simulink model "Final"  (R2019a)
settings: Solver=VariableStepAuto  StartTime=0.0  StopTime=100  RelTol=1e-3
undefined symbols (not defined in the file): sigbuilder_block
settings Model: Creator=fjvel  LastModifiedBy=fjvel

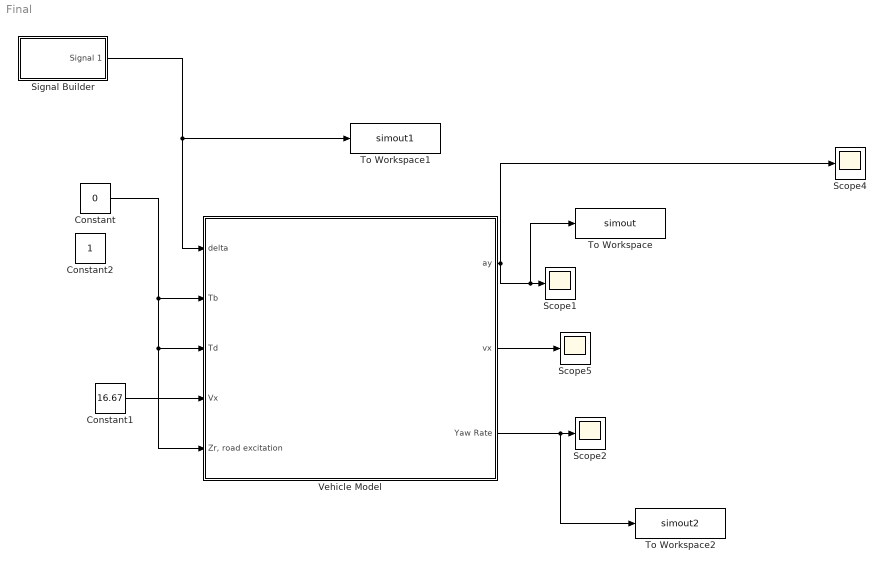
== system Final ==
  Constant : Constant  Value=0
  Constant1 : Constant  Value=16.67
  Constant2 : Constant
  Scope{1..2,4..5} (4 alike) : Scope
  Signal Builder : Subsystem  Tag=STV Subsys  LoadFcn=sigbuilder_block('load');  StartFcn=sigbuilder_block('start');  StopFcn=sigbuilder_block('stop');  ClipboardFcn=sigbuilder_block('clipboard');  mask(Sigbuilder block){tuvar=[0:10]}
      mask help: Simulink:masks:SigbuilderBlock_MD
      mask init:
      | if ~strcmp(get_param(bdroot(gcbh),'SimulationStatus'),'stopped') tuvar = sigbuilder_block('maskInit'); end
      settings: CopyFcn=sigbuilder_block('copy');  DeleteFcn=sigbuilder_block('delete');  ModelCloseFcn=sigbuilder_block('modelClose');  PreSaveFcn=sigbuilder_block('preSave');  PauseFcn=sigbuilder_block('pause');  ContinueFcn=sigbuilder_block('continue');  NameChangeFcn=sigbuilder_block('namechange');  OpenFcn=sigbuilder_block('open',[6 30 1012.5 447.75 ]);  CloseFcn=sigbuilder_block('close');
      mask Display: plot(0, 0, 100, 100,[2, 2, 32, 32, 2], [68, 8, 8, 68, 68],[32, 2], [38, 38], [32, 19, 2],[53, 60, 44], [32, 17, 17, 2],[16, 16, 31, 31]);txt = getActiveGroup(gcbh);text(2, 100, txt,'verticalAlignment', 'top');
  To Workspace : ToWorkspace  VariableName=simout  SaveFormat=Timeseries  SampleTime=-1
  To Workspace1 : ToWorkspace  VariableName=simout1  SaveFormat=Timeseries  SampleTime=-1
  To Workspace2 : ToWorkspace  VariableName=simout2  SaveFormat=Timeseries  SampleTime=-1
  Vehicle Model : Subsystem
  wires:
  Vehicle Model/2(vx) -> Scope5/1
  Constant/1 -> Vehicle Model/2(Tb), Vehicle Model/5("Zr, road excitation"), Vehicle Model/3(Td)
  Constant1/1 -> Vehicle Model/4("Vx ")
  Vehicle Model/1(ay) -> Scope4/1, To Workspace/1, Scope1/1
  Vehicle Model/3(Yaw Rate) -> To Workspace2/1, Scope2/1
  Signal Builder/1(Signal 1) -> Vehicle Model/1(delta), To Workspace1/1

== system Final/Signal Builder ==
  Demux : Demux  Tag=STV Demux  Outputs=1
  FromWs : FromWorkspace  Tag=STV FromWs  VariableName=tuvar  SampleTime=0
      SigBuilderData=|
      | common.afterFinalStr = 'Extrapolate'
      | common.sampleTime = 0
      | dataSet.timeRange = [0 10]
      | dataSet.name = 'Group 1'
      | sbobj.Groups.Name = 'Group 1'
      | sbobj.Groups.Signals.Name = 'Signal 1'
      | sbobj.Groups.Signals.XData = [0 3 3.03 3.47 3.5 10]
      | sbobj.Groups.Signals.YData = [0 0 0.042 0.042 0 0]
  Signal 1 : Outport  Tag=STV Outport
  wires:
  Demux/1 -> Signal 1/1
  FromWs/1 -> Demux/1

== system Final/Vehicle Model ==
  delta : Inport
  Tb : Inport  Port=2
  Td : Inport  Port=3
  "Vx " : Inport  Port=4  LockScale=on
  "Zr, road excitation" : Inport  Port=5
  Handling : Subsystem
  Scope : Scope
  Scope1 : Scope
  Scope2 : Scope
  Tire-Magic Formula Model : Subsystem
  Vertical Dynamics : Subsystem
  ay : Outport  VectorParamsAs1DForOutWhenUnconnected=on
  vx : Outport  Port=2  VectorParamsAs1DForOutWhenUnconnected=on
  Yaw Rate : Outport  Port=3  VectorParamsAs1DForOutWhenUnconnected=on
  wires:
  Handling/1(alpha_fl) -> Tire-Magic Formula Model/6(alpha_fl)
  Handling/2(alpha_fr) -> Tire-Magic Formula Model/8(alpha_fr)
  Handling/3(alpha_rl) -> Tire-Magic Formula Model/10(alpha_rl)
  Handling/4(alpha_rr) -> Tire-Magic Formula Model/12(alpha_rr)
  Handling/5(Sfl) -> Tire-Magic Formula Model/5(Sfl)
  Handling/6(Sfr) -> Tire-Magic Formula Model/7(Sfr)
  Handling/7(Srl) -> Tire-Magic Formula Model/9(Srl)
  Handling/8(Srr) -> Tire-Magic Formula Model/11(Srr)
  Tire-Magic Formula Model/1(Fxfl) -> Scope/1, Handling/2(Fxfl)
  Tire-Magic Formula Model/2(Fyfl) -> Scope1/1, Handling/3(Fyfl)
  Tire-Magic Formula Model/3(Fxfr) -> Handling/4(Fxfr)
  Tire-Magic Formula Model/4(Fyfr) -> Handling/5(Fyfr)
  Tire-Magic Formula Model/5(Fxrl) -> Handling/6(Fxrl)
  Tire-Magic Formula Model/6(Fyrl) -> Handling/7(Fyrl)
  Tire-Magic Formula Model/7(Fxrr) -> Handling/8(Fxrr)
  Tire-Magic Formula Model/8(Fyrr) -> Handling/9(Fyrr)
  Tire-Magic Formula Model/9(Mzfl) -> Scope2/1, Handling/10(Mzfl)
  Tire-Magic Formula Model/10(Mzfr) -> Handling/11(Mzfr)
  Tire-Magic Formula Model/11(Mzrl) -> Handling/12(Mzrl)
  Tire-Magic Formula Model/12(Mzrr) -> Handling/13(Mzrr)
  Td/1 -> Handling/14(Td)
  Tb/1 -> Handling/15(Tb)
  "Vx "/1 -> Handling/16(Vx)
  delta/1 -> Handling/1(delta)
  Handling/9(ax) -> Vertical Dynamics/1(ax)
  Handling/10(ay) -> ay/1, Vertical Dynamics/2(ay)
  Vertical Dynamics/1(Fzfl) -> Tire-Magic Formula Model/1(Fzfl)
  Vertical Dynamics/2(Fzfr) -> Tire-Magic Formula Model/2(Fzfr)
  Vertical Dynamics/3(Fzrl) -> Tire-Magic Formula Model/3("Fzrl ")
  Vertical Dynamics/4(Fzrr) -> Tire-Magic Formula Model/4(Fzrr)
  "Zr, road excitation"/1 -> Vertical Dynamics/3("Zr, road excitation")
  Handling/11("vx ") -> vx/1
  Handling/12(Yaw Rate) -> Yaw Rate/1

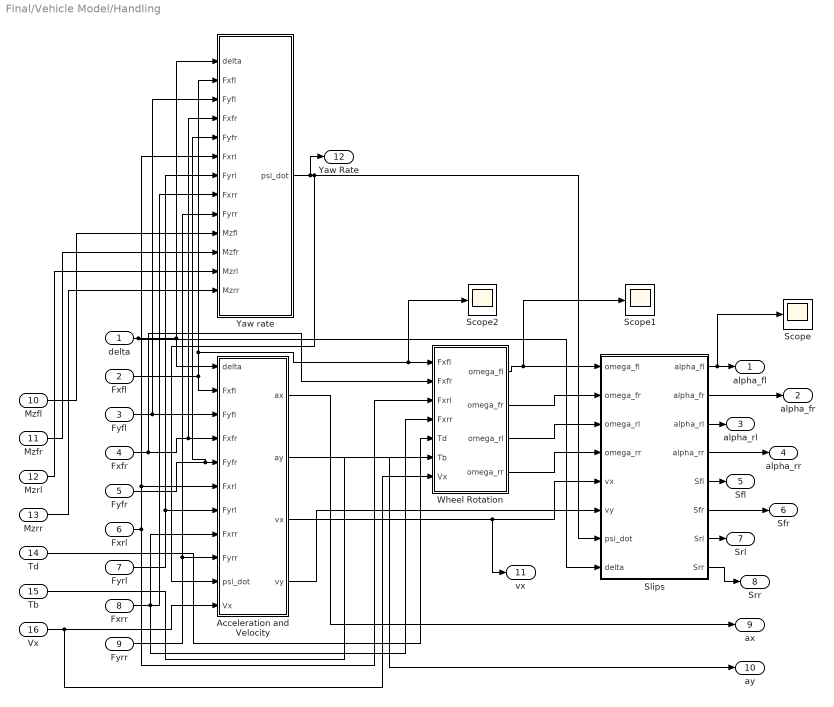
== system Final/Vehicle Model/Handling ==
  delta : Inport
  Fxfl : Inport  Port=2
  Fyfl : Inport  Port=3
  Fxfr : Inport  Port=4
  Fyfr : Inport  Port=5
  Fxrl : Inport  Port=6
  Fyrl : Inport  Port=7
  Fxrr : Inport  Port=8
  Fyrr : Inport  Port=9
  Mzfl : Inport  Port=10
  Mzfr : Inport  Port=11
  Mzrl : Inport  Port=12
  Mzrr : Inport  Port=13
  Td : Inport  Port=14
  Tb : Inport  Port=15
  Vx : Inport  Port=16
  "Acceleration and Velocity " : Subsystem
  Scope : Scope
  Scope1 : Scope
  Scope2 : Scope
  "Slips " : Subsystem
  Wheel Rotation : Subsystem
  Yaw rate : Subsystem
  alpha_fl : Outport
  alpha_fr : Outport  Port=2
  alpha_rl : Outport  Port=3
  alpha_rr : Outport  Port=4
  Sfl : Outport  Port=5
  Sfr : Outport  Port=6
  Srl : Outport  Port=7
  Srr : Outport  Port=8
  ax : Outport  Port=9
  ay : Outport  Port=10
  "vx " : Outport  Port=11  VectorParamsAs1DForOutWhenUnconnected=on
  Yaw Rate : Outport  Port=12  VectorParamsAs1DForOutWhenUnconnected=on
  wires:
  delta/1 -> "Slips "/8("delta "), Yaw rate/1(delta), "Acceleration and Velocity "/1(delta)
  Fxfl/1 -> Scope2/1, Wheel Rotation/1(Fxfl), Yaw rate/2(Fxfl), "Acceleration and Velocity "/2(Fxfl)
  Fyfl/1 -> Yaw rate/3(Fyfl), "Acceleration and Velocity "/3(Fyfl)
  Fxfr/1 -> Wheel Rotation/2(Fxfr), Yaw rate/4(Fxfr), "Acceleration and Velocity "/4(Fxfr)
  Fyfr/1 -> Yaw rate/5(Fyfr), "Acceleration and Velocity "/5(Fyfr)
  Fxrl/1 -> Wheel Rotation/3(Fxrl), Yaw rate/6(Fxrl), "Acceleration and Velocity "/6(Fxrl)
  Fyrl/1 -> Yaw rate/7(Fyrl), "Acceleration and Velocity "/7(Fyrl)
  Fxrr/1 -> Wheel Rotation/4(Fxrr), Yaw rate/8(Fxrr), "Acceleration and Velocity "/8(Fxrr)
  Fyrr/1 -> "Acceleration and Velocity "/9(Fyrr), Yaw rate/9(Fyrr)
  Vx/1 -> Wheel Rotation/7(Vx), "Acceleration and Velocity "/11(Vx)
  Mzfl/1 -> Yaw rate/10(Mzfl)
  Mzfr/1 -> Yaw rate/11(Mzfr)
  Mzrl/1 -> Yaw rate/12(Mzrl)
  Mzrr/1 -> Yaw rate/13(Mzrr)
  Yaw rate/1("psi_dot ") -> Yaw Rate/1, "Slips "/7(psi_dot), "Acceleration and Velocity "/10(psi_dot)
  Td/1 -> Wheel Rotation/5(Td)
  Tb/1 -> Wheel Rotation/6(Tb)
  Wheel Rotation/1(omega_fl) -> Scope1/1, "Slips "/1("omega_fl ")
  Wheel Rotation/2(omega_fr) -> "Slips "/2(omega_fr)
  Wheel Rotation/3(omega_rl) -> "Slips "/3(omega_rl)
  Wheel Rotation/4(omega_rr) -> "Slips "/4(omega_rr)
  "Acceleration and Velocity "/3(vx) -> "vx "/1, "Slips "/5(vx)
  "Acceleration and Velocity "/4(vy) -> "Slips "/6(vy)
  "Slips "/1(alpha_fl) -> Scope/1, alpha_fl/1
  "Slips "/2(alpha_fr) -> alpha_fr/1
  "Slips "/3(alpha_rl) -> alpha_rl/1
  "Slips "/4(alpha_rr) -> alpha_rr/1
  "Slips "/5("Sfl ") -> Sfl/1
  "Slips "/6(Sfr) -> Sfr/1
  "Slips "/7(Srl) -> Srl/1
  "Slips "/8(Srr) -> Srr/1
  "Acceleration and Velocity "/1(ax) -> ax/1
  "Acceleration and Velocity "/2(ay) -> ay/1

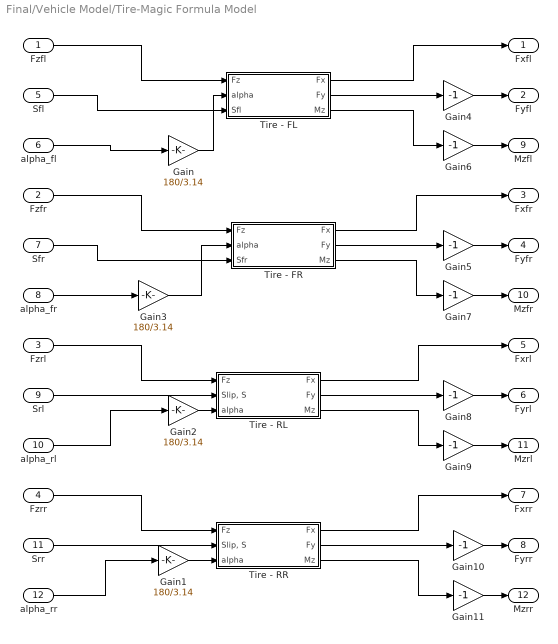
== system Final/Vehicle Model/Tire-Magic Formula Model ==
  Fzfl : Inport
  Fzfr : Inport  Port=2
  "Fzrl " : Inport  Port=3
  Fzrr : Inport  Port=4
  Sfl : Inport  Port=5
  alpha_fl : Inport  Port=6
  Sfr : Inport  Port=7
  alpha_fr : Inport  Port=8
  Srl : Inport  Port=9
  alpha_rl : Inport  Port=10
  Srr : Inport  Port=11
  alpha_rr : Inport  Port=12
  Gain{,1..3} (4 alike) : Gain  Gain=180/3.14
  Gain{4..11} (8 alike) : Gain  Gain=-1
  Tire - FL : Subsystem
  Tire - FR : Subsystem
  Tire - RL : Subsystem
  Tire - RR : Subsystem
  Fxfl : Outport
  Fyfl : Outport  Port=2
  Fxfr : Outport  Port=3
  Fyfr : Outport  Port=4
  Fxrl : Outport  Port=5
  Fyrl : Outport  Port=6
  Fxrr : Outport  Port=7
  Fyrr : Outport  Port=8
  Mzfl : Outport  Port=9
  Mzfr : Outport  Port=10
  Mzrl : Outport  Port=11
  Mzrr : Outport  Port=12
  wires:
  Fzfr/1 -> Tire - FR/1(Fz)
  Fzfl/1 -> Tire - FL/1(Fz)
  "Fzrl "/1 -> Tire - RL/1(Fz)
  Srl/1 -> Tire - RL/2("Slip, S")
  Fzrr/1 -> Tire - RR/1(Fz)
  Srr/1 -> Tire - RR/2("Slip, S")
  Tire - FL/1(Fx) -> Fxfl/1
  Tire - FL/2(Fy) -> Gain4/1
  Tire - FL/3(Mz) -> Gain6/1
  Tire - FR/2(Fy) -> Gain5/1
  Tire - FR/1(Fx) -> Fxfr/1
  Tire - FR/3(Mz) -> Gain7/1
  Tire - RL/1(Fx) -> Fxrl/1
  Tire - RL/2(Fy) -> Gain8/1
  Tire - RL/3(Mz) -> Gain9/1
  Tire - RR/1(Fx) -> Fxrr/1
  Tire - RR/2(Fy) -> Gain10/1
  Tire - RR/3(Mz) -> Gain11/1
  Sfl/1 -> Tire - FL/3("Sfl ")
  Sfr/1 -> Tire - FR/3(Sfr)
  alpha_fl/1 -> Gain/1
  Gain/1 -> Tire - FL/2(alpha)
  alpha_fr/1 -> Gain3/1
  Gain3/1 -> Tire - FR/2(alpha)
  Gain2/1 -> Tire - RL/3(alpha)
  Gain1/1 -> Tire - RR/3(alpha)
  alpha_rl/1 -> Gain2/1
  alpha_rr/1 -> Gain1/1
  Gain4/1 -> Fyfl/1
  Gain5/1 -> Fyfr/1
  Gain6/1 -> Mzfl/1
  Gain7/1 -> Mzfr/1
  Gain8/1 -> Fyrl/1
  Gain9/1 -> Mzrl/1
  Gain10/1 -> Fyrr/1
  Gain11/1 -> Mzrr/1

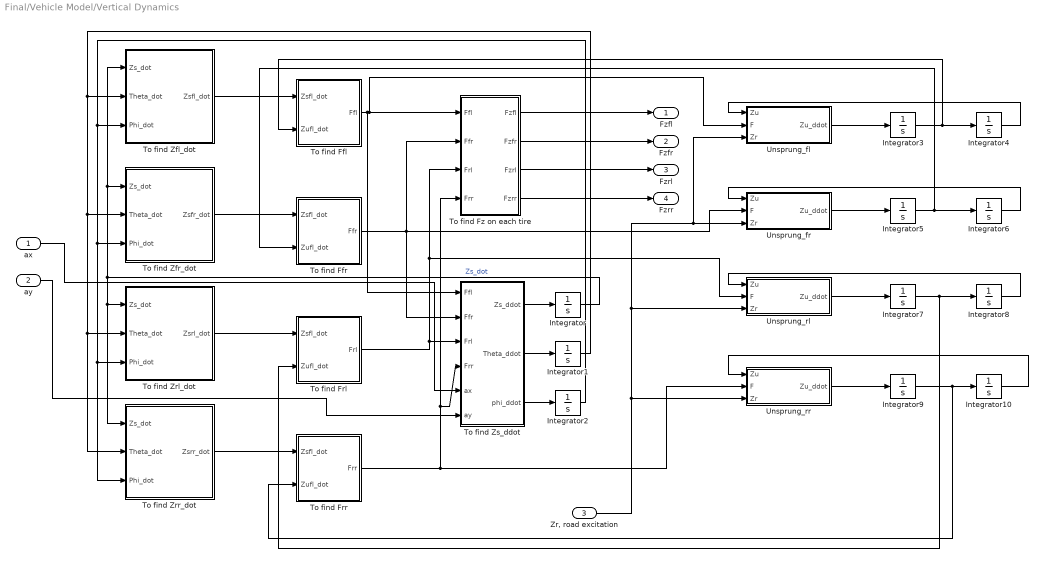
== system Final/Vehicle Model/Vertical Dynamics ==
  ax : Inport
  ay : Inport  Port=2
  "Zr, road excitation" : Inport  Port=3
  Integrator{,1..10} (11 alike) : Integrator
  "To find Ffl " : Subsystem
  To find Ffr : Subsystem
  To find Frl : Subsystem
  To find Frr : Subsystem
  To find Fz on each tire : Subsystem
  To find Zfl_dot : Subsystem
  To find Zfr_dot : Subsystem
  To find Zrl_dot : Subsystem
  To find Zrr_dot : Subsystem
  To find Zs_ddot : Subsystem
  Unsprung_fl : Subsystem
  Unsprung_fr : Subsystem
  Unsprung_rl : Subsystem
  Unsprung_rr : Subsystem
  Fzfl : Outport
  Fzfr : Outport  Port=2
  Fzrl : Outport  Port=3
  Fzrr : Outport  Port=4
  wires:
  To find Zfl_dot/1(Zsfl_dot) -> "To find Ffl "/1(Zsfl_dot)
  To find Zfr_dot/1(Zsfr_dot) -> To find Ffr/1(Zsfl_dot)
  To find Zrl_dot/1(Zsrl_dot) -> To find Frl/1(Zsfl_dot)
  To find Zrr_dot/1(Zsrr_dot) -> To find Frr/1(Zsfl_dot)
  "To find Ffl "/1(Ffl) -> To find Zs_ddot/1(Ffl), Unsprung_fl/2(F), To find Fz on each tire/1(Ffl)
  To find Ffr/1(Ffr) -> Unsprung_fr/2(F), To find Fz on each tire/2(Ffr), To find Zs_ddot/2(Ffr)
  To find Frl/1(Frl) -> Unsprung_rl/2(F), To find Fz on each tire/3(Frl), To find Zs_ddot/3(Frl)
  To find Frr/1(Frr) -> Unsprung_rr/2(F), To find Zs_ddot/4(Frr), To find Fz on each tire/4(Frr)
  To find Zs_ddot/1(Zs_ddot) -> Integrator/1
  Integrator/1 -> To find Zfl_dot/1(Zs_dot), To find Zfr_dot/1(Zs_dot), To find Zrr_dot/1(Zs_dot), To find Zrl_dot/1(Zs_dot)  "Zs_dot"
  To find Zs_ddot/2(Theta_ddot) -> Integrator1/1
  To find Zs_ddot/3(phi_ddot) -> Integrator2/1
  Integrator1/1 -> To find Zrr_dot/2(Theta_dot), To find Zrl_dot/2(Theta_dot), To find Zfr_dot/2(Theta_dot), To find Zfl_dot/2(Theta_dot)
  Integrator2/1 -> To find Zrr_dot/3(Phi_dot), To find Zrl_dot/3(Phi_dot), To find Zfr_dot/3(Phi_dot), To find Zfl_dot/3(Phi_dot)
  To find Fz on each tire/1(Fzfl) -> Fzfl/1
  To find Fz on each tire/2(Fzfr) -> Fzfr/1
  To find Fz on each tire/3(Fzrl) -> Fzrl/1
  To find Fz on each tire/4(Fzrr) -> Fzrr/1
  ax/1 -> To find Zs_ddot/5(ax)
  ay/1 -> To find Zs_ddot/6(ay)
  Integrator3/1 -> "To find Ffl "/2(Zufl_dot), Integrator4/1
  Unsprung_fl/1(Zu_ddot) -> Integrator3/1
  Integrator4/1 -> Unsprung_fl/1(Zu)
  Unsprung_fr/1(Zu_ddot) -> Integrator5/1
  Integrator5/1 -> To find Ffr/2(Zufl_dot), Integrator6/1
  Integrator6/1 -> Unsprung_fr/1(Zu)
  Unsprung_rl/1(Zu_ddot) -> Integrator7/1
  Integrator7/1 -> To find Frl/2(Zufl_dot), Integrator8/1
  Integrator8/1 -> Unsprung_rl/1(Zu)
  Unsprung_rr/1(Zu_ddot) -> Integrator9/1
  Integrator9/1 -> To find Frr/2(Zufl_dot), Integrator10/1
  Integrator10/1 -> Unsprung_rr/1(Zu)
  "Zr, road excitation"/1 -> Unsprung_fl/3(Zr), Unsprung_fr/3(Zr), Unsprung_rl/3(Zr), Unsprung_rr/3(Zr)

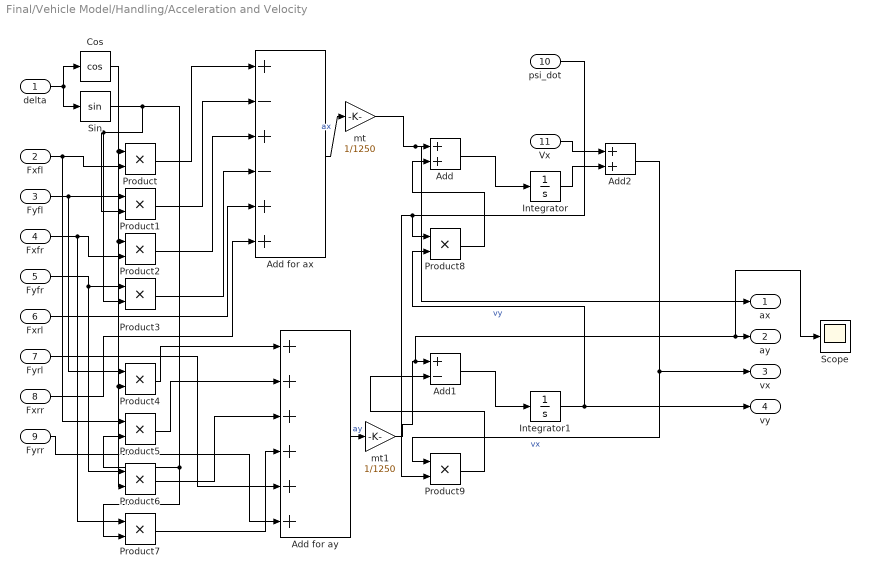
== system Final/Vehicle Model/Handling/Acceleration and Velocity  ==
  delta : Inport
  Fxfl : Inport  Port=2
  Fyfl : Inport  Port=3
  Fxfr : Inport  Port=4
  Fyfr : Inport  Port=5
  Fxrl : Inport  Port=6
  Fyrl : Inport  Port=7
  Fxrr : Inport  Port=8
  Fyrr : Inport  Port=9
  psi_dot : Inport  Port=10
  Vx : Inport  Port=11
  Add : Sum
  Add for ax : Sum  Inputs=+-+-++
  Add for ay : Sum  Inputs=++++++
  Add1 : Sum  Inputs=+-
  Add2 : Sum
  Cos : Trigonometry  Operator=cos
  Integrator : Integrator
  Integrator1 : Integrator
  Product{,1..9} (10 alike) : Product
  Scope : Scope
  Sin : Trigonometry
  mt : Gain  Gain=1/1250
  mt1 : Gain  Gain=1/1250
  ax : Outport
  ay : Outport  Port=2
  vx : Outport  Port=3
  vy : Outport  Port=4
  wires:
  delta/1 -> Sin/1, Cos/1
  Fxfl/1 -> Product5/1, Product/2
  Cos/1 -> Product6/2, Product4/2, Product2/1, Product/1
  Product/1 -> Add for ax/1
  Fyfl/1 -> Product4/1, Product1/1
  Sin/1 -> Product7/2, Product5/2, Product3/2, Product1/2
  Product1/1 -> Add for ax/2
  Fxfr/1 -> Product7/1, Product2/2
  Product2/1 -> Add for ax/3
  Fyfr/1 -> Product6/1, Product3/1
  Product3/1 -> Add for ax/4
  Fxrl/1 -> Add for ax/5
  Fxrr/1 -> Add for ax/6
  Product4/1 -> Add for ay/1
  Product5/1 -> Add for ay/2
  Product6/1 -> Add for ay/3
  Product7/1 -> Add for ay/4
  Fyrl/1 -> Add for ay/5
  Fyrr/1 -> Add for ay/6
  Add for ax/1 -> mt/1  "ax"
  Integrator1/1 -> vy/1, Product8/2  "vy"
  psi_dot/1 -> Product9/2, Product8/1
  Product8/1 -> Add/2
  Add/1 -> Integrator/1
  Product9/1 -> Add1/2
  Add1/1 -> Integrator1/1
  Vx/1 -> Add2/1
  Integrator/1 -> Add2/2
  Add2/1 -> vx/1, Product9/1  "vx"
  mt/1 -> ax/1, Add/1
  Add for ay/1 -> mt1/1  "ay"
  mt1/1 -> Scope/1, ay/1, Add1/1

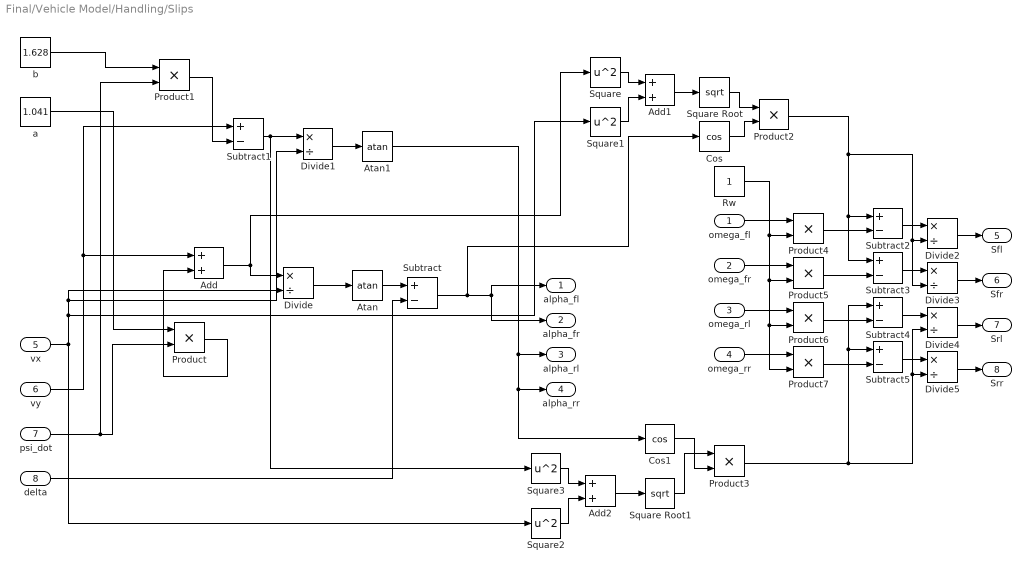
== system Final/Vehicle Model/Handling/Slips  ==
  "omega_fl " : Inport
  omega_fr : Inport  Port=2
  omega_rl : Inport  Port=3
  omega_rr : Inport  Port=4
  vx : Inport  Port=5
  vy : Inport  Port=6
  psi_dot : Inport  Port=7
  "delta " : Inport  Port=8
  Add : Sum
  Add1 : Sum
  Add2 : Sum
  Atan : Trigonometry  Operator=atan
  Atan1 : Trigonometry  Operator=atan
  Cos : Trigonometry  Operator=cos
  Cos1 : Trigonometry  Operator=cos
  Divide{,1..5} (6 alike) : Product  Inputs=*/
  Product{,1..7} (8 alike) : Product
  Rw : Constant
  Square{,1..3} (4 alike) : Math  Operator=square  SaturateOnIntegerOverflow=on
  Square Root : Sqrt  SaturateOnIntegerOverflow=on
  Square Root1 : Sqrt  SaturateOnIntegerOverflow=on
  Subtract{,1..5} (6 alike) : Sum  Inputs=+-
  a : Constant  Value=1.041
  b : Constant  Value=1.628
  alpha_fl : Outport
  alpha_fr : Outport  Port=2
  alpha_rl : Outport  Port=3
  alpha_rr : Outport  Port=4
  "Sfl " : Outport  Port=5
  Sfr : Outport  Port=6
  Srl : Outport  Port=7
  Srr : Outport  Port=8
  wires:
  psi_dot/1 -> Product1/2, Product/2
  a/1 -> Product/1
  vy/1 -> Subtract1/1, Add/1
  Product/1 -> Add/2
  Add/1 -> Square/1, Divide/1
  vx/1 -> Square2/1, Square1/1, Divide1/2, Divide/2
  Divide/1 -> Atan/1
  Atan/1 -> Subtract/1
  "delta "/1 -> Subtract/2
  Subtract/1 -> Cos/1, alpha_fr/1, alpha_fl/1
  b/1 -> Product1/1
  Product1/1 -> Subtract1/2
  Subtract1/1 -> Square3/1, Divide1/1
  Divide1/1 -> Atan1/1
  Atan1/1 -> Cos1/1, alpha_rr/1, alpha_rl/1
  Add1/1 -> Square Root/1
  Square/1 -> Add1/1
  Square1/1 -> Add1/2
  Add2/1 -> Square Root1/1
  Square3/1 -> Add2/1
  Square2/1 -> Add2/2
  Square Root/1 -> Product2/1
  Cos/1 -> Product2/2
  Cos1/1 -> Product3/2
  Square Root1/1 -> Product3/1
  omega_rr/1 -> Product7/1
  omega_rl/1 -> Product6/1
  omega_fr/1 -> Product5/1
  "omega_fl "/1 -> Product4/1
  Rw/1 -> Product7/2, Product6/2, Product5/2, Product4/2
  Product7/1 -> Subtract5/2
  Product6/1 -> Subtract4/2
  Product5/1 -> Subtract3/2
  Product4/1 -> Subtract2/2
  Product2/1 -> Divide3/2, Divide2/2, Subtract3/1, Subtract2/1
  Product3/1 -> Divide5/2, Divide4/2, Subtract4/1, Subtract5/1
  Subtract2/1 -> Divide2/1
  Subtract5/1 -> Divide5/1
  Subtract4/1 -> Divide4/1
  Subtract3/1 -> Divide3/1
  Divide5/1 -> Srr/1
  Divide4/1 -> Srl/1
  Divide3/1 -> Sfr/1
  Divide2/1 -> "Sfl "/1

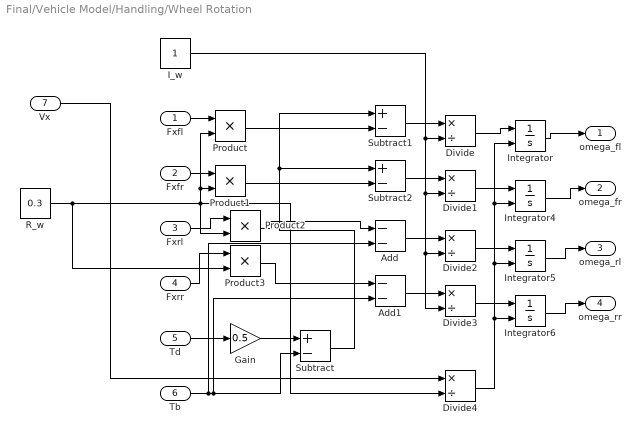
== system Final/Vehicle Model/Handling/Wheel Rotation ==
  Fxfl : Inport
  Fxfr : Inport  Port=2
  Fxrl : Inport  Port=3
  Fxrr : Inport  Port=4
  Td : Inport  Port=5
  Tb : Inport  Port=6
  Vx : Inport  Port=7
  Add : Sum  Inputs=--
  Add1 : Sum  Inputs=--
  Divide{,1..4} (5 alike) : Product  Inputs=*/
  Gain : Gain  Gain=0.5
  I_w : Constant
  Integrator{,4..6} (4 alike) : Integrator  InitialConditionSource=external
  Product{,1..3} (4 alike) : Product
  R_w : Constant  Value=0.3
  Subtract : Sum  Inputs=+-
  Subtract1 : Sum  Inputs=+-
  Subtract2 : Sum  Inputs=+-
  omega_fl : Outport
  omega_fr : Outport  Port=2
  omega_rl : Outport  Port=3
  omega_rr : Outport  Port=4
  wires:
  Td/1 -> Gain/1
  Fxfl/1 -> Product/1
  R_w/1 -> Product3/2, Product2/2, Divide4/2, Product1/2, Product/2
  Gain/1 -> Subtract/1
  Tb/1 -> Add/2, Add1/2, Subtract/2
  Product/1 -> Subtract1/2
  Subtract/1 -> Subtract2/1, Subtract1/1
  Fxfr/1 -> Product1/1
  Product1/1 -> Subtract2/2
  Subtract1/1 -> Divide/1
  Subtract2/1 -> Divide1/1
  Add/1 -> Divide2/1
  Add1/1 -> Divide3/1
  I_w/1 -> Divide3/2, Divide2/2, Divide1/2, Divide/2
  Divide/1 -> Integrator/1
  Divide1/1 -> Integrator4/1
  Divide2/1 -> Integrator5/1
  Divide3/1 -> Integrator6/1
  Integrator5/1 -> omega_rl/1
  Integrator6/1 -> omega_rr/1
  Integrator4/1 -> omega_fr/1
  Integrator/1 -> omega_fl/1
  Vx/1 -> Divide4/1
  Divide4/1 -> Integrator6/2, Integrator5/2, Integrator/2, Integrator4/2
  Fxrl/1 -> Product2/1
  Product2/1 -> Add/1
  Product3/1 -> Add1/1
  Fxrr/1 -> Product3/1

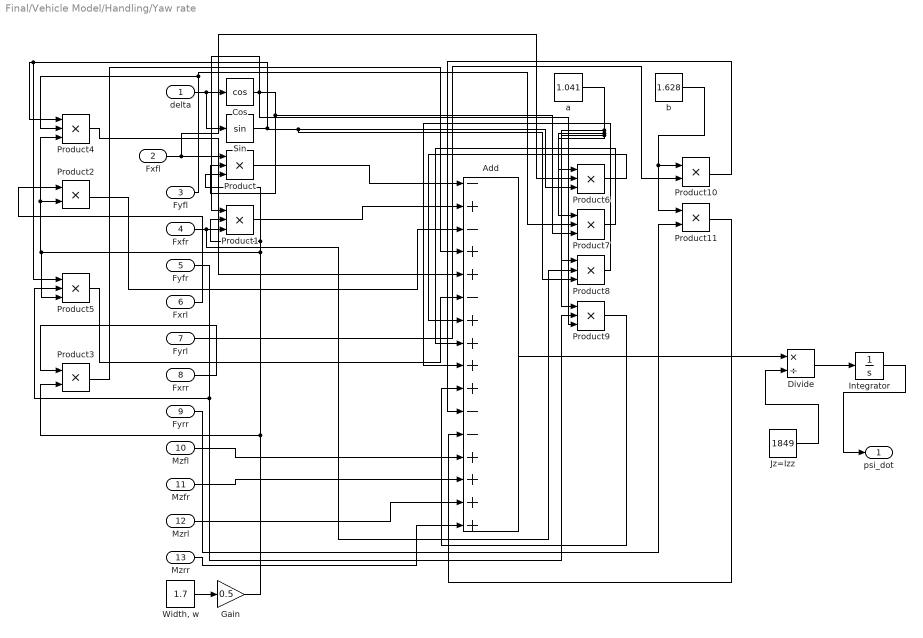
== system Final/Vehicle Model/Handling/Yaw rate ==
  delta : Inport
  Fxfl : Inport  Port=2
  Fyfl : Inport  Port=3
  Fxfr : Inport  Port=4
  Fyfr : Inport  Port=5
  Fxrl : Inport  Port=6
  Fyrl : Inport  Port=7
  Fxrr : Inport  Port=8
  Fyrr : Inport  Port=9
  Mzfl : Inport  Port=10
  Mzfr : Inport  Port=11
  Mzrl : Inport  Port=12
  Mzrr : Inport  Port=13
  Add : Sum  Inputs=-+-++-++++--++++
  Cos : Trigonometry  Operator=cos
  Divide : Product  Inputs=*/
  Gain : Gain  Gain=0.5
  Integrator : Integrator
  Jz=Izz : Constant  Value=1849
  Product{,1,4..9} (8 alike) : Product  Inputs=3
  Product{2..3,10..11} (4 alike) : Product
  Sin : Trigonometry
  "Width, w" : Constant  Value=1.7
  a : Constant  Value=1.041
  b : Constant  Value=1.628
  "psi_dot " : Outport
  wires:
  delta/1 -> Sin/1, Cos/1
  "Width, w"/1 -> Gain/1
  Fxfl/1 -> Product6/2, Product/1
  Cos/1 -> Product9/3, Product1/1, Product7/3, Product/2
  Gain/1 -> Product5/3, Product4/3, Product2/2, Product1/2, Product/3, Product3/2
  Product/1 -> Add/1
  Fxfr/1 -> Product8/2, Product1/3
  Product1/1 -> Add/2
  Fxrl/1 -> Product2/1
  Product2/1 -> Add/3
  Fxrr/1 -> Product3/1
  Product3/1 -> Add/4
  Fyfl/1 -> Product7/2, Product4/2
  Sin/1 -> Product8/3, Product6/3, Product5/1, Product4/1
  Product4/1 -> Add/5
  Fyfr/1 -> Product9/2, Product5/2
  Product5/1 -> Add/6
  a/1 -> Product9/1, Product6/1, Product7/1, Product8/1
  Product6/1 -> Add/7
  Product7/1 -> Add/8
  Product8/1 -> Add/9
  Product9/1 -> Add/10
  b/1 -> Product11/1, Product10/1
  Fyrl/1 -> Product10/2
  Product10/1 -> Add/11
  Fyrr/1 -> Product11/2
  Product11/1 -> Add/12
  Mzfl/1 -> Add/13
  Mzfr/1 -> Add/14
  Mzrl/1 -> Add/15
  Mzrr/1 -> Add/16
  Add/1 -> Divide/1
  Jz=Izz/1 -> Divide/2
  Divide/1 -> Integrator/1
  Integrator/1 -> "psi_dot "/1

== system Final/Vehicle Model/Tire-Magic Formula Model/Tire - FL ==
  Fz : Inport
  alpha : Inport  Port=2
  "Sfl " : Inport  Port=3
  Sub_Fx : Subsystem
  Sub_Fy : Subsystem
  Sub_Mz : Subsystem
  Fx : Outport
  Fy : Outport  Port=2
  Mz : Outport  Port=3
  wires:
  Fz/1 -> Sub_Fx/1(Fz), Sub_Mz/1(Fz), Sub_Fy/1(Fz)
  alpha/1 -> Sub_Mz/2(alpha), Sub_Fy/2(alpha)
  Sub_Fx/1(F) -> Fx/1
  Sub_Fy/1(F) -> Fy/1
  Sub_Mz/1(F) -> Mz/1
  "Sfl "/1 -> Sub_Fx/2(Slip)

== system Final/Vehicle Model/Tire-Magic Formula Model/Tire - FR ==
  Fz : Inport
  alpha : Inport  Port=2
  Sfr : Inport  Port=3
  Sub_Fx : Subsystem
  Sub_Fy : Subsystem
  Sub_Mz : Subsystem
  Fx : Outport
  Fy : Outport  Port=2
  Mz : Outport  Port=3
  wires:
  Fz/1 -> Sub_Mz/1(Fz), Sub_Fy/1(Fz), Sub_Fx/1(Fz)
  alpha/1 -> Sub_Mz/2(alpha), Sub_Fy/2(alpha)
  Sub_Fx/1(F) -> Fx/1
  Sub_Fy/1(F) -> Fy/1
  Sub_Mz/1(F) -> Mz/1
  Sfr/1 -> Sub_Fx/2(Slip)

== system Final/Vehicle Model/Tire-Magic Formula Model/Tire - RL ==
  Fz : Inport
  "Slip, S" : Inport  Port=2
  alpha : Inport  Port=3
  Sub_Fx : Subsystem
  Sub_Fy : Subsystem
  Sub_Mz : Subsystem
  Fx : Outport
  Fy : Outport  Port=2
  Mz : Outport  Port=3
  wires:
  Fz/1 -> Sub_Mz/1(Fz), Sub_Fy/1(Fz), Sub_Fx/1(Fz)
  alpha/1 -> Sub_Mz/2(alpha), Sub_Fy/2(alpha)
  Sub_Fx/1(F) -> Fx/1
  Sub_Fy/1(F) -> Fy/1
  Sub_Mz/1(F) -> Mz/1
  "Slip, S"/1 -> Sub_Fx/2(Slip)

== system Final/Vehicle Model/Tire-Magic Formula Model/Tire - RR ==
  Fz : Inport
  "Slip, S" : Inport  Port=2
  alpha : Inport  Port=3
  Sub_Fx : Subsystem
  Sub_Fy : Subsystem
  Sub_Mz : Subsystem
  Fx : Outport
  Fy : Outport  Port=2
  Mz : Outport  Port=3
  wires:
  Fz/1 -> Sub_Mz/1(Fz), Sub_Fy/1(Fz), Sub_Fx/1(Fz)
  alpha/1 -> Sub_Mz/2(alpha), Sub_Fy/2(alpha)
  Sub_Fx/1(F) -> Fx/1
  Sub_Fy/1(F) -> Fy/1
  Sub_Mz/1(F) -> Mz/1
  "Slip, S"/1 -> Sub_Fx/2(Slip)

== system Final/Vehicle Model/Vertical Dynamics/To find Ffl  ==
  Zsfl_dot : Inport
  Zufl_dot : Inport  Port=2
  Add : Sum
  C : Gain  Gain=1600
  Integrator : Integrator
  Integrator1 : Integrator
  K : Gain  Gain=25000
  Subtract : Sum  Inputs=-+
  Subtract1 : Sum  Inputs=-+
  Ffl : Outport
  wires:
  Zsfl_dot/1 -> Integrator/1, Subtract/1
  Zufl_dot/1 -> Integrator1/1, Subtract/2
  Integrator/1 -> Subtract1/1
  Integrator1/1 -> Subtract1/2
  Subtract/1 -> C/1
  Subtract1/1 -> K/1
  C/1 -> Add/1
  K/1 -> Add/2
  Add/1 -> Ffl/1

== system Final/Vehicle Model/Vertical Dynamics/To find Ffr ==
  Zsfl_dot : Inport
  Zufl_dot : Inport  Port=2
  Add : Sum
  C : Gain  Gain=1600
  Integrator : Integrator
  Integrator1 : Integrator
  K : Gain  Gain=25000
  Subtract : Sum  Inputs=-+
  Subtract1 : Sum  Inputs=-+
  Ffr : Outport
  wires:
  Zsfl_dot/1 -> Integrator/1, Subtract/1
  Zufl_dot/1 -> Integrator1/1, Subtract/2
  Integrator/1 -> Subtract1/1
  Integrator1/1 -> Subtract1/2
  Subtract/1 -> C/1
  Subtract1/1 -> K/1
  C/1 -> Add/1
  K/1 -> Add/2
  Add/1 -> Ffr/1

== system Final/Vehicle Model/Vertical Dynamics/To find Frl ==
  Zsfl_dot : Inport
  Zufl_dot : Inport  Port=2
  Add : Sum
  C : Gain  Gain=2000
  Integrator : Integrator
  Integrator1 : Integrator
  K : Gain  Gain=30000
  Subtract : Sum  Inputs=-+
  Subtract1 : Sum  Inputs=-+
  Frl : Outport
  wires:
  Zsfl_dot/1 -> Integrator/1, Subtract/1
  Zufl_dot/1 -> Integrator1/1, Subtract/2
  Integrator/1 -> Subtract1/1
  Integrator1/1 -> Subtract1/2
  Subtract/1 -> C/1
  Subtract1/1 -> K/1
  C/1 -> Add/1
  K/1 -> Add/2
  Add/1 -> Frl/1

== system Final/Vehicle Model/Vertical Dynamics/To find Frr ==
  Zsfl_dot : Inport
  Zufl_dot : Inport  Port=2
  Add : Sum
  C : Gain  Gain=2000
  Integrator : Integrator
  Integrator1 : Integrator
  K : Gain  Gain=30000
  Subtract : Sum  Inputs=-+
  Subtract1 : Sum  Inputs=-+
  Frr : Outport
  wires:
  Zsfl_dot/1 -> Integrator/1, Subtract/1
  Zufl_dot/1 -> Integrator1/1, Subtract/2
  Integrator/1 -> Subtract1/1
  Integrator1/1 -> Subtract1/2
  Subtract/1 -> C/1
  Subtract1/1 -> K/1
  C/1 -> Add/1
  K/1 -> Add/2
  Add/1 -> Frr/1

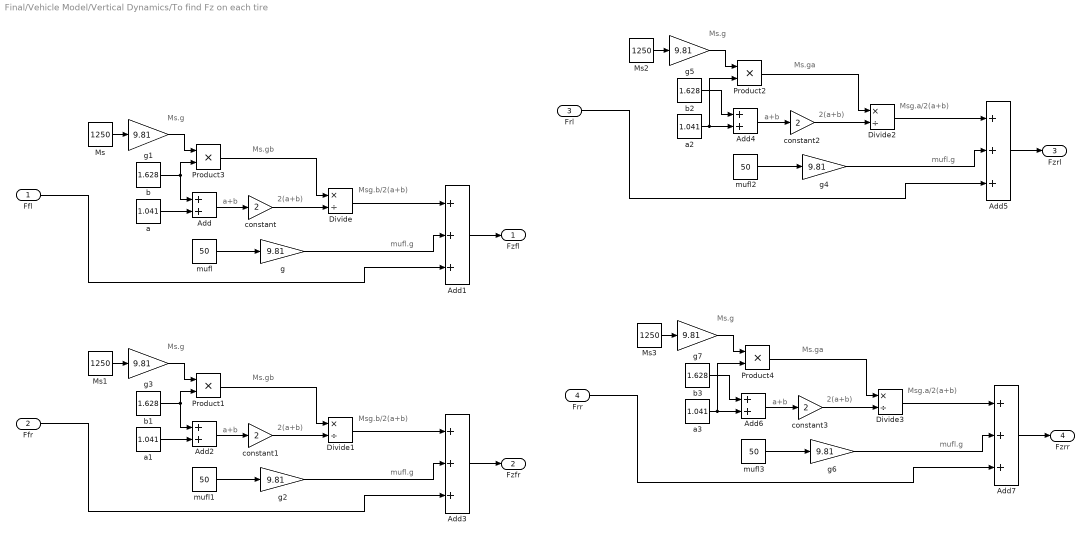
== system Final/Vehicle Model/Vertical Dynamics/To find Fz on each tire ==
  note: Ms.g
  note: Ms.gb
  note: a+b
  note: Msg.b/2(a+b)
  note: mufl.g
  note: 2(a+b)
  note: Msg.b/2(a+b)
  note: Ms.gb
  note: 2(a+b)
  note: a+b
  note: Ms.g
  note: mufl.g
  note: Msg.a/2(a+b)
  note: Ms.ga
  note: 2(a+b)
  note: a+b
  note: Ms.g
  note: mufl.g
  note: Ms.g
  note: mufl.g
  note: Msg.a/2(a+b)
  note: Ms.ga
  note: 2(a+b)
  note: a+b
  Ffl : Inport
  Ffr : Inport  Port=2
  Frl : Inport  Port=3
  Frr : Inport  Port=4
  Add{,2,4,6} (4 alike) : Sum
  Add{1,3,5,7} (4 alike) : Sum  Inputs=+++
  Divide{,1..3} (4 alike) : Product  Inputs=*/
  Ms{,1..3} (4 alike) : Constant  Value=1250
  Product{1..4} (4 alike) : Product  RndMeth=Zero
  a{,1..3} (4 alike) : Constant  Value=1.041
  b{,1..3} (4 alike) : Constant  Value=1.628
  constant{,1..3} (4 alike) : Gain  Gain=2
  g{,1..7} (8 alike) : Gain  Gain=9.81
  mufl{,1..3} (4 alike) : Constant  Value=50
  Fzfl : Outport
  Fzfr : Outport  Port=2
  Fzrl : Outport  Port=3
  Fzrr : Outport  Port=4
  wires:
  Ffl/1 -> Add1/3
  constant/1 -> Divide/2
  Add/1 -> constant/1
  g1/1 -> Product3/1
  mufl/1 -> g/1
  Product3/1 -> Divide/1
  Ms/1 -> g1/1
  g/1 -> Add1/2
  b/1 -> Product3/2, Add/1
  a/1 -> Add/2
  Divide/1 -> Add1/1
  Add1/1 -> Fzfl/1
  Product1/1 -> Divide1/1
  mufl1/1 -> g2/1
  g3/1 -> Product1/1
  Add3/1 -> Fzfr/1
  constant1/1 -> Divide1/2
  Add2/1 -> constant1/1
  g2/1 -> Add3/2
  a1/1 -> Add2/2
  Divide1/1 -> Add3/1
  Ms1/1 -> g3/1
  Ffr/1 -> Add3/3
  b1/1 -> Product1/2, Add2/1
  Product2/1 -> Divide2/1
  mufl2/1 -> g4/1
  g5/1 -> Product2/1
  Add5/1 -> Fzrl/1
  constant2/1 -> Divide2/2
  Add4/1 -> constant2/1
  g4/1 -> Add5/2
  a2/1 -> Product2/2, Add4/2
  Divide2/1 -> Add5/1
  Ms2/1 -> g5/1
  Frl/1 -> Add5/3
  b2/1 -> Add4/1
  b3/1 -> Add6/1
  a3/1 -> Product4/2, Add6/2
  Ms3/1 -> g7/1
  Frr/1 -> Add7/3
  g6/1 -> Add7/2
  mufl3/1 -> g6/1
  g7/1 -> Product4/1
  Divide3/1 -> Add7/1
  Add6/1 -> constant3/1
  constant3/1 -> Divide3/2
  Product4/1 -> Divide3/1
  Add7/1 -> Fzrr/1

== system Final/Vehicle Model/Vertical Dynamics/To find Zfl_dot ==
  Zs_dot : Inport
  Theta_dot : Inport  Port=2
  Phi_dot : Inport  Port=3
  Add : Sum  Inputs=+-+
  a : Gain  Gain=1.041
  w/2 : Gain  Gain=0.85
  Zsfl_dot : Outport
  wires:
  Zs_dot/1 -> Add/1
  Theta_dot/1 -> a/1
  a/1 -> Add/2
  w/2/1 -> Add/3
  Phi_dot/1 -> w/2/1
  Add/1 -> Zsfl_dot/1

== system Final/Vehicle Model/Vertical Dynamics/To find Zfr_dot ==
  Zs_dot : Inport
  Theta_dot : Inport  Port=2
  Phi_dot : Inport  Port=3
  Add : Sum  Inputs=+--
  a : Gain  Gain=1.041
  w/2 : Gain  Gain=0.85
  Zsfr_dot : Outport
  wires:
  Zs_dot/1 -> Add/1
  Theta_dot/1 -> a/1
  a/1 -> Add/2
  w/2/1 -> Add/3
  Phi_dot/1 -> w/2/1
  Add/1 -> Zsfr_dot/1

== system Final/Vehicle Model/Vertical Dynamics/To find Zrl_dot ==
  Zs_dot : Inport
  Theta_dot : Inport  Port=2
  Phi_dot : Inport  Port=3
  Add : Sum  Inputs=+++
  b : Gain  Gain=1.628
  w/2 : Gain  Gain=0.85
  Zsrl_dot : Outport
  wires:
  Zs_dot/1 -> Add/1
  Theta_dot/1 -> b/1
  b/1 -> Add/2
  w/2/1 -> Add/3
  Phi_dot/1 -> w/2/1
  Add/1 -> Zsrl_dot/1

== system Final/Vehicle Model/Vertical Dynamics/To find Zrr_dot ==
  Zs_dot : Inport
  Theta_dot : Inport  Port=2
  Phi_dot : Inport  Port=3
  Add : Sum  Inputs=++-
  b : Gain  Gain=1.628
  w/2 : Gain  Gain=0.85
  Zsrr_dot : Outport
  wires:
  Zs_dot/1 -> Add/1
  Theta_dot/1 -> b/1
  b/1 -> Add/2
  w/2/1 -> Add/3
  Phi_dot/1 -> w/2/1
  Add/1 -> Zsrr_dot/1

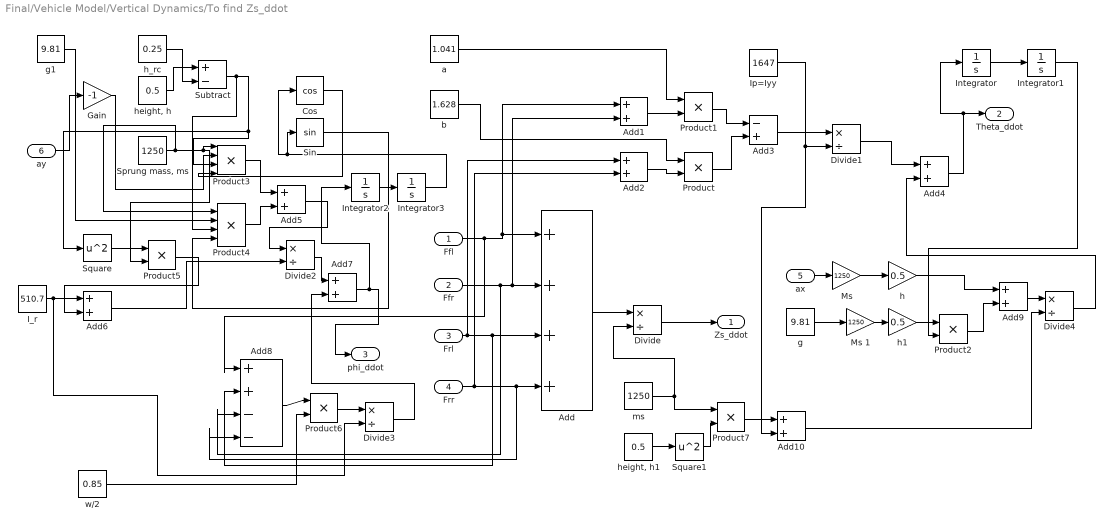
== system Final/Vehicle Model/Vertical Dynamics/To find Zs_ddot ==
  Ffl : Inport
  Ffr : Inport  Port=2
  Frl : Inport  Port=3
  Frr : Inport  Port=4
  ax : Inport  Port=5
  ay : Inport  Port=6
  Add : Sum  Inputs=++++
  Add{1..2,4..7,9..10} (8 alike) : Sum
  Add3 : Sum  Inputs=-+
  Add8 : Sum  Inputs=++--
  Cos : Trigonometry  Operator=cos
  Divide{,1..4} (5 alike) : Product  Inputs=*/
  Gain : Gain  Gain=-1
  I_r : Constant  Value=510.7
  Integrator{,1..3} (4 alike) : Integrator
  Ip=Iyy : Constant  Value=1647
  "Ms " : Gain  Gain=1250
  Ms 1 : Gain  Gain=1250
  Product{,1..2,5..7} (6 alike) : Product
  Product3 : Product  Inputs=4
  Product4 : Product  Inputs=4
  Sin : Trigonometry
  "Sprung mass, ms" : Constant  Value=1250
  Square : Math  Operator=square  SaturateOnIntegerOverflow=on
  Square1 : Math  Operator=square  SaturateOnIntegerOverflow=on
  Subtract : Sum  Inputs=+-
  "a " : Constant  Value=1.041
  b : Constant  Value=1.628
  g : Constant  Value=9.81
  g1 : Constant  Value=9.81
  h : Gain  Gain=0.5
  h1 : Gain  Gain=0.5
  h_rc : Constant  Value=0.25
  "height, h" : Constant  Value=0.5
  "height, h1" : Constant  Value=0.5
  ms : Constant  Value=1250
  "w/2 " : Constant  Value=0.85
  Zs_ddot : Outport
  Theta_ddot : Outport  Port=2
  phi_ddot : Outport  Port=3
  wires:
  Frr/1 -> Add2/2, Add8/4, Add/4
  Frl/1 -> Add2/1, Add8/2, Add/3
  Ffr/1 -> Add8/3, Add1/2, Add/2
  Ffl/1 -> Add8/1, Add1/1, Add/1
  Add/1 -> Divide/1
  ms/1 -> Product7/1, Divide/2
  Divide/1 -> Zs_ddot/1
  Add2/1 -> Product/2
  b/1 -> Product/1
  "a "/1 -> Product1/1
  Add1/1 -> Product1/2
  Product1/1 -> Add3/1
  Product/1 -> Add3/2
  Add3/1 -> Divide1/1
  Ip=Iyy/1 -> Add10/2, Divide1/2
  Divide1/1 -> Add4/1
  Add4/1 -> Integrator/1, Theta_ddot/1
  ax/1 -> "Ms "/1
  "Ms "/1 -> h/1
  g/1 -> Ms 1/1
  Ms 1/1 -> h1/1
  h1/1 -> Product2/1
  Integrator/1 -> Integrator1/1
  Integrator1/1 -> Product2/2
  h_rc/1 -> Subtract/2
  "height, h"/1 -> Subtract/1
  "Sprung mass, ms"/1 -> Product5/2, Product3/1, Product4/1
  Subtract/1 -> Product4/3, Square/1, Product3/3
  g1/1 -> Product4/2
  Product3/1 -> Add5/1
  Product4/1 -> Add5/2
  Add5/1 -> Divide2/1
  Square/1 -> Product5/1
  Product5/1 -> Add6/2
  Add6/1 -> Divide2/2
  Divide2/1 -> Add7/1
  Add7/1 -> Integrator2/1, phi_ddot/1
  Integrator2/1 -> Integrator3/1
  Integrator3/1 -> Sin/1, Cos/1
  Cos/1 -> Product3/4
  Sin/1 -> Product4/4
  Add8/1 -> Product6/1
  "w/2 "/1 -> Product6/2
  Product6/1 -> Divide3/1
  I_r/1 -> Divide3/2, Add6/1
  Divide3/1 -> Add7/2
  h/1 -> Add9/1
  Product2/1 -> Add9/2
  Add9/1 -> Divide4/1
  Add10/1 -> Divide4/2
  Divide4/1 -> Add4/2
  "height, h1"/1 -> Square1/1
  Square1/1 -> Product7/2
  Product7/1 -> Add10/1
  ay/1 -> Gain/1
  Gain/1 -> Product3/2

== system Final/Vehicle Model/Vertical Dynamics/Unsprung_fl ==
  Zu : Inport
  F : Inport  Port=2
  Zr : Inport  Port=3
  Divide : Product  Inputs=*/
  K_tire : Gain  Gain=100000
  Subtract : Sum  Inputs=+-
  Subtract1 : Sum  Inputs=+-
  "Unsprung mass, mu" : Constant  Value=50
  Zu_ddot : Outport
  wires:
  Zr/1 -> Subtract/1
  Zu/1 -> Subtract/2
  Subtract/1 -> K_tire/1
  K_tire/1 -> Subtract1/1
  F/1 -> Subtract1/2
  Subtract1/1 -> Divide/1
  Divide/1 -> Zu_ddot/1
  "Unsprung mass, mu"/1 -> Divide/2

== system Final/Vehicle Model/Vertical Dynamics/Unsprung_fr ==
  Zu : Inport
  F : Inport  Port=2
  Zr : Inport  Port=3
  Divide : Product  Inputs=*/
  K_tire : Gain  Gain=100000
  Subtract : Sum  Inputs=+-
  Subtract1 : Sum  Inputs=+-
  "Unsprung mass, mu" : Constant  Value=50
  Zu_ddot : Outport
  wires:
  Zr/1 -> Subtract/1
  Zu/1 -> Subtract/2
  Subtract/1 -> K_tire/1
  K_tire/1 -> Subtract1/1
  F/1 -> Subtract1/2
  Subtract1/1 -> Divide/1
  Divide/1 -> Zu_ddot/1
  "Unsprung mass, mu"/1 -> Divide/2

== system Final/Vehicle Model/Vertical Dynamics/Unsprung_rl ==
  Zu : Inport
  F : Inport  Port=2
  Zr : Inport  Port=3
  Divide : Product  Inputs=*/
  K_tire : Gain  Gain=100000
  Subtract : Sum  Inputs=+-
  Subtract1 : Sum  Inputs=+-
  "Unsprung mass, mu" : Constant  Value=50
  Zu_ddot : Outport
  wires:
  Zr/1 -> Subtract/1
  Zu/1 -> Subtract/2
  Subtract/1 -> K_tire/1
  K_tire/1 -> Subtract1/1
  F/1 -> Subtract1/2
  Subtract1/1 -> Divide/1
  Divide/1 -> Zu_ddot/1
  "Unsprung mass, mu"/1 -> Divide/2

== system Final/Vehicle Model/Vertical Dynamics/Unsprung_rr ==
  Zu : Inport
  F : Inport  Port=2
  Zr : Inport  Port=3
  Divide : Product  Inputs=*/
  K_tire : Gain  Gain=100000
  Subtract : Sum  Inputs=+-
  Subtract1 : Sum  Inputs=+-
  "Unsprung mass, mu" : Constant  Value=50
  Zu_ddot : Outport
  wires:
  Zr/1 -> Subtract/1
  Zu/1 -> Subtract/2
  Subtract/1 -> K_tire/1
  K_tire/1 -> Subtract1/1
  F/1 -> Subtract1/2
  Subtract1/1 -> Divide/1
  Divide/1 -> Zu_ddot/1
  "Unsprung mass, mu"/1 -> Divide/2

== system Final/Vehicle Model/Tire-Magic Formula Model/Tire - FL/Sub_Fx ==
  Fz : Inport
  Slip : Inport  Port=2
  B : Constant  Value=24.12
  C : Constant  Value=0.501
  D : Constant  Value=2.088
  E : Constant  Value=1.027
  Subsystem : Subsystem
  F : Outport
  wires:
  Fz/1 -> Subsystem/1(Fz)
  Slip/1 -> Subsystem/2(x)
  Subsystem/1("F/M ") -> F/1
  E/1 -> Subsystem/6(E)
  D/1 -> Subsystem/5(D)
  C/1 -> Subsystem/4(C)
  B/1 -> Subsystem/3(B)

== system Final/Vehicle Model/Tire-Magic Formula Model/Tire - FL/Sub_Fy ==
  Fz : Inport
  alpha : Inport  Port=2
  B : Constant  Value=0.1506
  C : Constant  Value=1.351
  D : Constant  Value=0.8846
  E : Constant  Value=-1.883
  Subsystem : Subsystem
  F : Outport
  wires:
  Fz/1 -> Subsystem/1(Fz)
  alpha/1 -> Subsystem/2(x)
  Subsystem/1("F/M ") -> F/1
  E/1 -> Subsystem/6(E)
  D/1 -> Subsystem/5(D)
  C/1 -> Subsystem/4(C)
  B/1 -> Subsystem/3(B)

== system Final/Vehicle Model/Tire-Magic Formula Model/Tire - FL/Sub_Mz ==
  Fz : Inport
  alpha : Inport  Port=2
  B : Constant  Value=0.1874
  C : Constant  Value=-2.204
  D : Constant  Value=-0.02117
  E : Constant  Value=-3.308
  Subsystem : Subsystem
  F : Outport
  wires:
  Fz/1 -> Subsystem/1(Fz)
  alpha/1 -> Subsystem/2(x)
  Subsystem/1("F/M ") -> F/1
  E/1 -> Subsystem/6(E)
  D/1 -> Subsystem/5(D)
  C/1 -> Subsystem/4(C)
  B/1 -> Subsystem/3(B)

== system Final/Vehicle Model/Tire-Magic Formula Model/Tire - FR/Sub_Fx ==
  Fz : Inport
  Slip : Inport  Port=2
  B : Constant  Value=24.12
  C : Constant  Value=0.501
  D : Constant  Value=2.088
  E : Constant  Value=1.027
  Subsystem : Subsystem
  F : Outport
  wires:
  Fz/1 -> Subsystem/1(Fz)
  Slip/1 -> Subsystem/2(x)
  Subsystem/1("F/M ") -> F/1
  E/1 -> Subsystem/6(E)
  D/1 -> Subsystem/5(D)
  C/1 -> Subsystem/4(C)
  B/1 -> Subsystem/3(B)

== system Final/Vehicle Model/Tire-Magic Formula Model/Tire - FR/Sub_Fy ==
  Fz : Inport
  alpha : Inport  Port=2
  B : Constant  Value=0.1506
  C : Constant  Value=1.351
  D : Constant  Value=0.8846
  E : Constant  Value=-1.883
  Subsystem : Subsystem
  F : Outport
  wires:
  Fz/1 -> Subsystem/1(Fz)
  alpha/1 -> Subsystem/2(x)
  Subsystem/1("F/M ") -> F/1
  E/1 -> Subsystem/6(E)
  D/1 -> Subsystem/5(D)
  C/1 -> Subsystem/4(C)
  B/1 -> Subsystem/3(B)

== system Final/Vehicle Model/Tire-Magic Formula Model/Tire - FR/Sub_Mz ==
  Fz : Inport
  alpha : Inport  Port=2
  B : Constant  Value=0.1874
  C : Constant  Value=-2.204
  D : Constant  Value=-0.02117
  E : Constant  Value=-3.308
  Subsystem : Subsystem
  F : Outport
  wires:
  Fz/1 -> Subsystem/1(Fz)
  alpha/1 -> Subsystem/2(x)
  Subsystem/1("F/M ") -> F/1
  E/1 -> Subsystem/6(E)
  D/1 -> Subsystem/5(D)
  C/1 -> Subsystem/4(C)
  B/1 -> Subsystem/3(B)

== system Final/Vehicle Model/Tire-Magic Formula Model/Tire - RL/Sub_Fx ==
  Fz : Inport
  Slip : Inport  Port=2
  B : Constant  Value=24.12
  C : Constant  Value=0.501
  D : Constant  Value=2.088
  E : Constant  Value=1.027
  Subsystem : Subsystem
  F : Outport
  wires:
  Fz/1 -> Subsystem/1(Fz)
  Slip/1 -> Subsystem/2(x)
  Subsystem/1("F/M ") -> F/1
  E/1 -> Subsystem/6(E)
  D/1 -> Subsystem/5(D)
  C/1 -> Subsystem/4(C)
  B/1 -> Subsystem/3(B)

== system Final/Vehicle Model/Tire-Magic Formula Model/Tire - RL/Sub_Fy ==
  Fz : Inport
  alpha : Inport  Port=2
  B : Constant  Value=0.1506
  C : Constant  Value=1.351
  D : Constant  Value=0.8846
  E : Constant  Value=-1.883
  Subsystem : Subsystem
  F : Outport
  wires:
  Fz/1 -> Subsystem/1(Fz)
  alpha/1 -> Subsystem/2(x)
  Subsystem/1("F/M ") -> F/1
  E/1 -> Subsystem/6(E)
  D/1 -> Subsystem/5(D)
  C/1 -> Subsystem/4(C)
  B/1 -> Subsystem/3(B)

== system Final/Vehicle Model/Tire-Magic Formula Model/Tire - RL/Sub_Mz ==
  Fz : Inport
  alpha : Inport  Port=2
  B : Constant  Value=0.1874
  C : Constant  Value=-2.204
  D : Constant  Value=-0.02117
  E : Constant  Value=-3.308
  Subsystem : Subsystem
  F : Outport
  wires:
  Fz/1 -> Subsystem/1(Fz)
  alpha/1 -> Subsystem/2(x)
  Subsystem/1("F/M ") -> F/1
  E/1 -> Subsystem/6(E)
  D/1 -> Subsystem/5(D)
  C/1 -> Subsystem/4(C)
  B/1 -> Subsystem/3(B)

== system Final/Vehicle Model/Tire-Magic Formula Model/Tire - RR/Sub_Fx ==
  Fz : Inport
  Slip : Inport  Port=2
  B : Constant  Value=24.12
  C : Constant  Value=0.501
  D : Constant  Value=2.088
  E : Constant  Value=1.027
  Subsystem : Subsystem
  F : Outport
  wires:
  Fz/1 -> Subsystem/1(Fz)
  Slip/1 -> Subsystem/2(x)
  Subsystem/1("F/M ") -> F/1
  E/1 -> Subsystem/6(E)
  D/1 -> Subsystem/5(D)
  C/1 -> Subsystem/4(C)
  B/1 -> Subsystem/3(B)

== system Final/Vehicle Model/Tire-Magic Formula Model/Tire - RR/Sub_Fy ==
  Fz : Inport
  alpha : Inport  Port=2
  B : Constant  Value=0.1506
  C : Constant  Value=1.351
  D : Constant  Value=0.8846
  E : Constant  Value=-1.883
  Subsystem : Subsystem
  F : Outport
  wires:
  Fz/1 -> Subsystem/1(Fz)
  alpha/1 -> Subsystem/2(x)
  Subsystem/1("F/M ") -> F/1
  E/1 -> Subsystem/6(E)
  D/1 -> Subsystem/5(D)
  C/1 -> Subsystem/4(C)
  B/1 -> Subsystem/3(B)

== system Final/Vehicle Model/Tire-Magic Formula Model/Tire - RR/Sub_Mz ==
  Fz : Inport
  alpha : Inport  Port=2
  B : Constant  Value=0.1874
  C : Constant  Value=-2.204
  D : Constant  Value=-0.02117
  E : Constant  Value=-3.308
  Subsystem : Subsystem
  F : Outport
  wires:
  Fz/1 -> Subsystem/1(Fz)
  alpha/1 -> Subsystem/2(x)
  Subsystem/1("F/M ") -> F/1
  E/1 -> Subsystem/6(E)
  D/1 -> Subsystem/5(D)
  C/1 -> Subsystem/4(C)
  B/1 -> Subsystem/3(B)

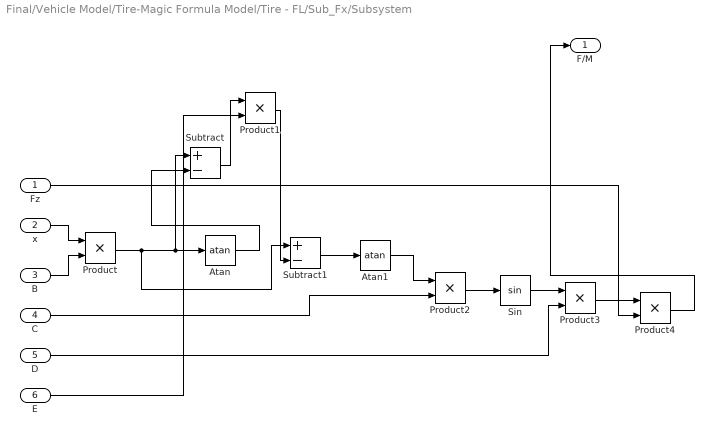
== system Final/Vehicle Model/Tire-Magic Formula Model/Tire - FL/Sub_Fx/Subsystem ==
  Fz : Inport
  x : Inport  Port=2
  B : Inport  Port=3
  C : Inport  Port=4
  D : Inport  Port=5
  E : Inport  Port=6
  Atan : Trigonometry  Operator=atan
  Atan1 : Trigonometry  Operator=atan
  Product{,1..4} (5 alike) : Product
  Sin : Trigonometry
  Subtract : Sum  Inputs=+-
  Subtract1 : Sum  Inputs=+-
  "F/M " : Outport
  wires:
  x/1 -> Product/1
  B/1 -> Product/2
  Product/1 -> Subtract1/1, Subtract/1, Atan/1
  Atan/1 -> Subtract/2
  E/1 -> Product1/2
  Subtract/1 -> Product1/1
  Product1/1 -> Subtract1/2
  Subtract1/1 -> Atan1/1
  Atan1/1 -> Product2/1
  C/1 -> Product2/2
  Product2/1 -> Sin/1
  Sin/1 -> Product3/1
  D/1 -> Product3/2
  Product3/1 -> Product4/1
  Fz/1 -> Product4/2
  Product4/1 -> "F/M "/1

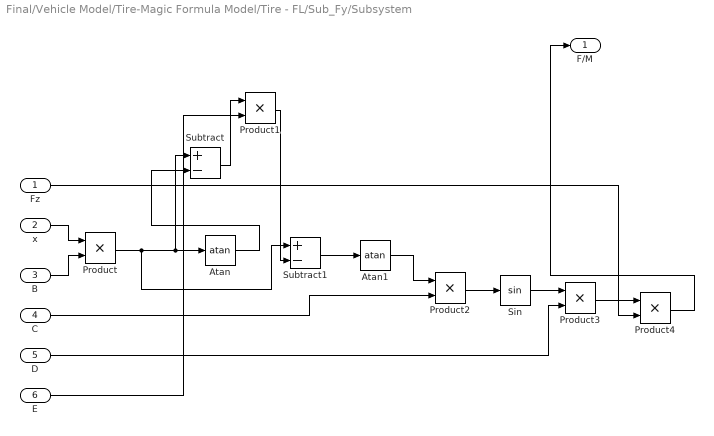
== system Final/Vehicle Model/Tire-Magic Formula Model/Tire - FL/Sub_Fy/Subsystem ==
  Fz : Inport
  x : Inport  Port=2
  B : Inport  Port=3
  C : Inport  Port=4
  D : Inport  Port=5
  E : Inport  Port=6
  Atan : Trigonometry  Operator=atan
  Atan1 : Trigonometry  Operator=atan
  Product{,1..4} (5 alike) : Product
  Sin : Trigonometry
  Subtract : Sum  Inputs=+-
  Subtract1 : Sum  Inputs=+-
  "F/M " : Outport
  wires:
  x/1 -> Product/1
  B/1 -> Product/2
  Product/1 -> Subtract1/1, Subtract/1, Atan/1
  Atan/1 -> Subtract/2
  E/1 -> Product1/2
  Subtract/1 -> Product1/1
  Product1/1 -> Subtract1/2
  Subtract1/1 -> Atan1/1
  Atan1/1 -> Product2/1
  C/1 -> Product2/2
  Product2/1 -> Sin/1
  Sin/1 -> Product3/1
  D/1 -> Product3/2
  Product3/1 -> Product4/1
  Fz/1 -> Product4/2
  Product4/1 -> "F/M "/1

== system Final/Vehicle Model/Tire-Magic Formula Model/Tire - FL/Sub_Mz/Subsystem ==
  Fz : Inport
  x : Inport  Port=2
  B : Inport  Port=3
  C : Inport  Port=4
  D : Inport  Port=5
  E : Inport  Port=6
  Atan : Trigonometry  Operator=atan
  Atan1 : Trigonometry  Operator=atan
  Product{,1..4} (5 alike) : Product
  Sin : Trigonometry
  Subtract : Sum  Inputs=+-
  Subtract1 : Sum  Inputs=+-
  "F/M " : Outport
  wires:
  x/1 -> Product/1
  B/1 -> Product/2
  Product/1 -> Subtract1/1, Subtract/1, Atan/1
  Atan/1 -> Subtract/2
  E/1 -> Product1/2
  Subtract/1 -> Product1/1
  Product1/1 -> Subtract1/2
  Subtract1/1 -> Atan1/1
  Atan1/1 -> Product2/1
  C/1 -> Product2/2
  Product2/1 -> Sin/1
  Sin/1 -> Product3/1
  D/1 -> Product3/2
  Product3/1 -> Product4/1
  Fz/1 -> Product4/2
  Product4/1 -> "F/M "/1

== system Final/Vehicle Model/Tire-Magic Formula Model/Tire - FR/Sub_Fx/Subsystem ==
  Fz : Inport
  x : Inport  Port=2
  B : Inport  Port=3
  C : Inport  Port=4
  D : Inport  Port=5
  E : Inport  Port=6
  Atan : Trigonometry  Operator=atan
  Atan1 : Trigonometry  Operator=atan
  Product{,1..4} (5 alike) : Product
  Sin : Trigonometry
  Subtract : Sum  Inputs=+-
  Subtract1 : Sum  Inputs=+-
  "F/M " : Outport
  wires:
  x/1 -> Product/1
  B/1 -> Product/2
  Product/1 -> Subtract/1, Atan/1, Subtract1/1
  Atan/1 -> Subtract/2
  E/1 -> Product1/2
  Subtract/1 -> Product1/1
  Product1/1 -> Subtract1/2
  Subtract1/1 -> Atan1/1
  Atan1/1 -> Product2/1
  C/1 -> Product2/2
  Product2/1 -> Sin/1
  Sin/1 -> Product3/1
  D/1 -> Product3/2
  Product3/1 -> Product4/1
  Fz/1 -> Product4/2
  Product4/1 -> "F/M "/1

== system Final/Vehicle Model/Tire-Magic Formula Model/Tire - FR/Sub_Fy/Subsystem ==
  Fz : Inport
  x : Inport  Port=2
  B : Inport  Port=3
  C : Inport  Port=4
  D : Inport  Port=5
  E : Inport  Port=6
  Atan : Trigonometry  Operator=atan
  Atan1 : Trigonometry  Operator=atan
  Product{,1..4} (5 alike) : Product
  Sin : Trigonometry
  Subtract : Sum  Inputs=+-
  Subtract1 : Sum  Inputs=+-
  "F/M " : Outport
  wires:
  x/1 -> Product/1
  B/1 -> Product/2
  Product/1 -> Subtract1/1, Subtract/1, Atan/1
  Atan/1 -> Subtract/2
  E/1 -> Product1/2
  Subtract/1 -> Product1/1
  Product1/1 -> Subtract1/2
  Subtract1/1 -> Atan1/1
  Atan1/1 -> Product2/1
  C/1 -> Product2/2
  Product2/1 -> Sin/1
  Sin/1 -> Product3/1
  D/1 -> Product3/2
  Product3/1 -> Product4/1
  Fz/1 -> Product4/2
  Product4/1 -> "F/M "/1

== system Final/Vehicle Model/Tire-Magic Formula Model/Tire - FR/Sub_Mz/Subsystem ==
  Fz : Inport
  x : Inport  Port=2
  B : Inport  Port=3
  C : Inport  Port=4
  D : Inport  Port=5
  E : Inport  Port=6
  Atan : Trigonometry  Operator=atan
  Atan1 : Trigonometry  Operator=atan
  Product{,1..4} (5 alike) : Product
  Sin : Trigonometry
  Subtract : Sum  Inputs=+-
  Subtract1 : Sum  Inputs=+-
  "F/M " : Outport
  wires:
  x/1 -> Product/1
  B/1 -> Product/2
  Product/1 -> Subtract1/1, Subtract/1, Atan/1
  Atan/1 -> Subtract/2
  E/1 -> Product1/2
  Subtract/1 -> Product1/1
  Product1/1 -> Subtract1/2
  Subtract1/1 -> Atan1/1
  Atan1/1 -> Product2/1
  C/1 -> Product2/2
  Product2/1 -> Sin/1
  Sin/1 -> Product3/1
  D/1 -> Product3/2
  Product3/1 -> Product4/1
  Fz/1 -> Product4/2
  Product4/1 -> "F/M "/1

== system Final/Vehicle Model/Tire-Magic Formula Model/Tire - RL/Sub_Fx/Subsystem ==
  Fz : Inport
  x : Inport  Port=2
  B : Inport  Port=3
  C : Inport  Port=4
  D : Inport  Port=5
  E : Inport  Port=6
  Atan : Trigonometry  Operator=atan
  Atan1 : Trigonometry  Operator=atan
  Product{,1..4} (5 alike) : Product
  Sin : Trigonometry
  Subtract : Sum  Inputs=+-
  Subtract1 : Sum  Inputs=+-
  "F/M " : Outport
  wires:
  x/1 -> Product/1
  B/1 -> Product/2
  Product/1 -> Subtract1/1, Subtract/1, Atan/1
  Atan/1 -> Subtract/2
  E/1 -> Product1/2
  Subtract/1 -> Product1/1
  Product1/1 -> Subtract1/2
  Subtract1/1 -> Atan1/1
  Atan1/1 -> Product2/1
  C/1 -> Product2/2
  Product2/1 -> Sin/1
  Sin/1 -> Product3/1
  D/1 -> Product3/2
  Product3/1 -> Product4/1
  Fz/1 -> Product4/2
  Product4/1 -> "F/M "/1

== system Final/Vehicle Model/Tire-Magic Formula Model/Tire - RL/Sub_Fy/Subsystem ==
  Fz : Inport
  x : Inport  Port=2
  B : Inport  Port=3
  C : Inport  Port=4
  D : Inport  Port=5
  E : Inport  Port=6
  Atan : Trigonometry  Operator=atan
  Atan1 : Trigonometry  Operator=atan
  Product{,1..4} (5 alike) : Product
  Sin : Trigonometry
  Subtract : Sum  Inputs=+-
  Subtract1 : Sum  Inputs=+-
  "F/M " : Outport
  wires:
  x/1 -> Product/1
  B/1 -> Product/2
  Product/1 -> Subtract1/1, Subtract/1, Atan/1
  Atan/1 -> Subtract/2
  E/1 -> Product1/2
  Subtract/1 -> Product1/1
  Product1/1 -> Subtract1/2
  Subtract1/1 -> Atan1/1
  Atan1/1 -> Product2/1
  C/1 -> Product2/2
  Product2/1 -> Sin/1
  Sin/1 -> Product3/1
  D/1 -> Product3/2
  Product3/1 -> Product4/1
  Fz/1 -> Product4/2
  Product4/1 -> "F/M "/1

== system Final/Vehicle Model/Tire-Magic Formula Model/Tire - RL/Sub_Mz/Subsystem ==
  Fz : Inport
  x : Inport  Port=2
  B : Inport  Port=3
  C : Inport  Port=4
  D : Inport  Port=5
  E : Inport  Port=6
  Atan : Trigonometry  Operator=atan
  Atan1 : Trigonometry  Operator=atan
  Product{,1..4} (5 alike) : Product
  Sin : Trigonometry
  Subtract : Sum  Inputs=+-
  Subtract1 : Sum  Inputs=+-
  "F/M " : Outport
  wires:
  x/1 -> Product/1
  B/1 -> Product/2
  Product/1 -> Subtract1/1, Subtract/1, Atan/1
  Atan/1 -> Subtract/2
  E/1 -> Product1/2
  Subtract/1 -> Product1/1
  Product1/1 -> Subtract1/2
  Subtract1/1 -> Atan1/1
  Atan1/1 -> Product2/1
  C/1 -> Product2/2
  Product2/1 -> Sin/1
  Sin/1 -> Product3/1
  D/1 -> Product3/2
  Product3/1 -> Product4/1
  Fz/1 -> Product4/2
  Product4/1 -> "F/M "/1

== system Final/Vehicle Model/Tire-Magic Formula Model/Tire - RR/Sub_Fx/Subsystem ==
  Fz : Inport
  x : Inport  Port=2
  B : Inport  Port=3
  C : Inport  Port=4
  D : Inport  Port=5
  E : Inport  Port=6
  Atan : Trigonometry  Operator=atan
  Atan1 : Trigonometry  Operator=atan
  Product{,1..4} (5 alike) : Product
  Sin : Trigonometry
  Subtract : Sum  Inputs=+-
  Subtract1 : Sum  Inputs=+-
  "F/M " : Outport
  wires:
  x/1 -> Product/1
  B/1 -> Product/2
  Product/1 -> Subtract1/1, Subtract/1, Atan/1
  Atan/1 -> Subtract/2
  E/1 -> Product1/2
  Subtract/1 -> Product1/1
  Product1/1 -> Subtract1/2
  Subtract1/1 -> Atan1/1
  Atan1/1 -> Product2/1
  C/1 -> Product2/2
  Product2/1 -> Sin/1
  Sin/1 -> Product3/1
  D/1 -> Product3/2
  Product3/1 -> Product4/1
  Fz/1 -> Product4/2
  Product4/1 -> "F/M "/1

== system Final/Vehicle Model/Tire-Magic Formula Model/Tire - RR/Sub_Fy/Subsystem ==
  Fz : Inport
  x : Inport  Port=2
  B : Inport  Port=3
  C : Inport  Port=4
  D : Inport  Port=5
  E : Inport  Port=6
  Atan : Trigonometry  Operator=atan
  Atan1 : Trigonometry  Operator=atan
  Product{,1..4} (5 alike) : Product
  Sin : Trigonometry
  Subtract : Sum  Inputs=+-
  Subtract1 : Sum  Inputs=+-
  "F/M " : Outport
  wires:
  x/1 -> Product/1
  B/1 -> Product/2
  Product/1 -> Subtract1/1, Subtract/1, Atan/1
  Atan/1 -> Subtract/2
  E/1 -> Product1/2
  Subtract/1 -> Product1/1
  Product1/1 -> Subtract1/2
  Subtract1/1 -> Atan1/1
  Atan1/1 -> Product2/1
  C/1 -> Product2/2
  Product2/1 -> Sin/1
  Sin/1 -> Product3/1
  D/1 -> Product3/2
  Product3/1 -> Product4/1
  Fz/1 -> Product4/2
  Product4/1 -> "F/M "/1

== system Final/Vehicle Model/Tire-Magic Formula Model/Tire - RR/Sub_Mz/Subsystem ==
  Fz : Inport
  x : Inport  Port=2
  B : Inport  Port=3
  C : Inport  Port=4
  D : Inport  Port=5
  E : Inport  Port=6
  Atan : Trigonometry  Operator=atan
  Atan1 : Trigonometry  Operator=atan
  Product{,1..4} (5 alike) : Product
  Sin : Trigonometry
  Subtract : Sum  Inputs=+-
  Subtract1 : Sum  Inputs=+-
  "F/M " : Outport
  wires:
  x/1 -> Product/1
  B/1 -> Product/2
  Product/1 -> Subtract1/1, Subtract/1, Atan/1
  Atan/1 -> Subtract/2
  E/1 -> Product1/2
  Subtract/1 -> Product1/1
  Product1/1 -> Subtract1/2
  Subtract1/1 -> Atan1/1
  Atan1/1 -> Product2/1
  C/1 -> Product2/2
  Product2/1 -> Sin/1
  Sin/1 -> Product3/1
  D/1 -> Product3/2
  Product3/1 -> Product4/1
  Fz/1 -> Product4/2
  Product4/1 -> "F/M "/1
